simulink model "part2"  (R2018a)
settings: Solver=VariableStepAuto  StartTime=0.0  StopTime=2.9  RelTol=1e-3
libraries: truetime x1
settings Model: Creator=Ismael  LastModifiedBy=Ismael

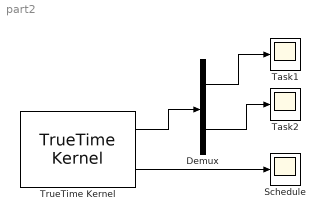
== system part2 ==
  Demux : Demux  Outputs=2
  Schedule : Scope
  "Task1 " : Scope
  Task2 : Scope
  TrueTime Kernel : truetime/TrueTime Kernel  sfun=part2_init  args=1  ninputsoutputs=[0 2]  ntriggers=0  trigtype=falling  nwnodenbr=[]  clockoffsetdrift=[0 0]  schedoutput=on  battery=off  poweroutput=off
  wires:
  TrueTime Kernel/1 -> Demux/1
  Demux/1 -> "Task1 "/1
  Demux/2 -> Task2/1
  TrueTime Kernel/2 -> Schedule/1
